simulink model "sim12ex8"  (Simulink 4.00)
settings: Solver=ode45  SolverMode=SingleTasking  StartTime=0.0  StopTime=2  MaxStep=.010  RelTol=1e-3  AbsTol=1e-3
libraries: simulink_extras x1
settings Model: LastModifiedBy=saadat  SaveTime=off  SaveOutput=off  LimitDataPoints=off  RTWTemplateMakefile=grt_vc.tmf  ExtModeTrigMode=oneshot  ExtModeArmWhenConnect=off

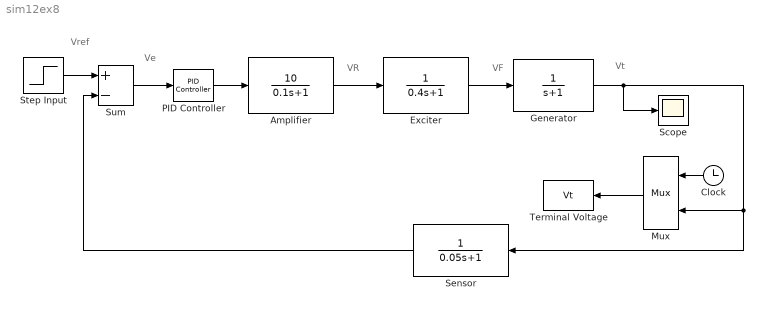
== system sim12ex8 ==
  note: Ve
  note: Vt
  note: VF
  note: VR
  note: Vref
  Amplifier : TransferFcn  Numerator=10  Denominator="[0.1  1]"  AbsoluteTolerance=auto  Realization=auto
  Clock : Clock
      settings: DisplayTime=off  Decimation=10
  Exciter : TransferFcn  Numerator=1  Denominator="[0.4  1]"  AbsoluteTolerance=auto  Realization=auto
  Generator : TransferFcn  Numerator=[1]  Denominator="[1  1]"  AbsoluteTolerance=auto  Realization=auto
  Mux : Mux  Orientation=left  Inputs=2
      settings: DisplayOption=none
  PID Controller : simulink_extras/Additional Linear/PID Controller  P=1  I=0.25  D=0.28
  Scope : Scope
      settings: TickLabels=on  TimeRange=2  YMin=0  YMax=1.5  SaveToWorkspace=off  SaveName=ScopeData  DataFormat=Array  LimitDataPoints=on  MaxDataPoints=5000
  Sensor : TransferFcn  Orientation=left  Numerator=[1]  Denominator="[0.05  1]"  AbsoluteTolerance=auto  Realization=auto
  Step Input : Step  Time=0  Before=1  After=1  SampleTime=0
  Sum : Sum  Inputs=+-  SaturateOnIntegerOverflow=on
  Terminal Voltage : ToWorkspace  VariableName=Vt  SampleTime=0  SaveFormat=Array
      settings: MaxDataPoints=1000
  wires:
  Generator/1 -> Scope/1, Mux/2, Sensor/1
  Clock/1 -> Mux/1
  Mux/1 -> Terminal Voltage/1
  PID Controller/1 -> Amplifier/1
  Sum/1 -> PID Controller/1
  Amplifier/1 -> Exciter/1
  Sensor/1 -> Sum/2
  Exciter/1 -> Generator/1
  Step Input/1 -> Sum/1
